simulink model "MMA"  (R2022a)
settings: Solver=VariableStepAuto  StartTime=0.0  StopTime=10.0  FixedStep=Ts  RelTol=1e-3
settings Model: Creator=juani  LastModifiedBy=juani

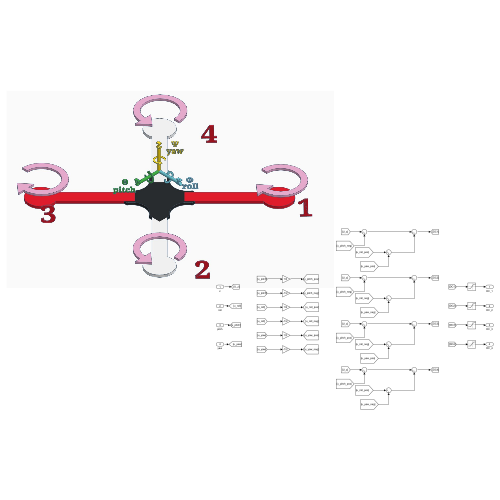
[thumbnail: Simulink's stored preview of the top-level diagram]
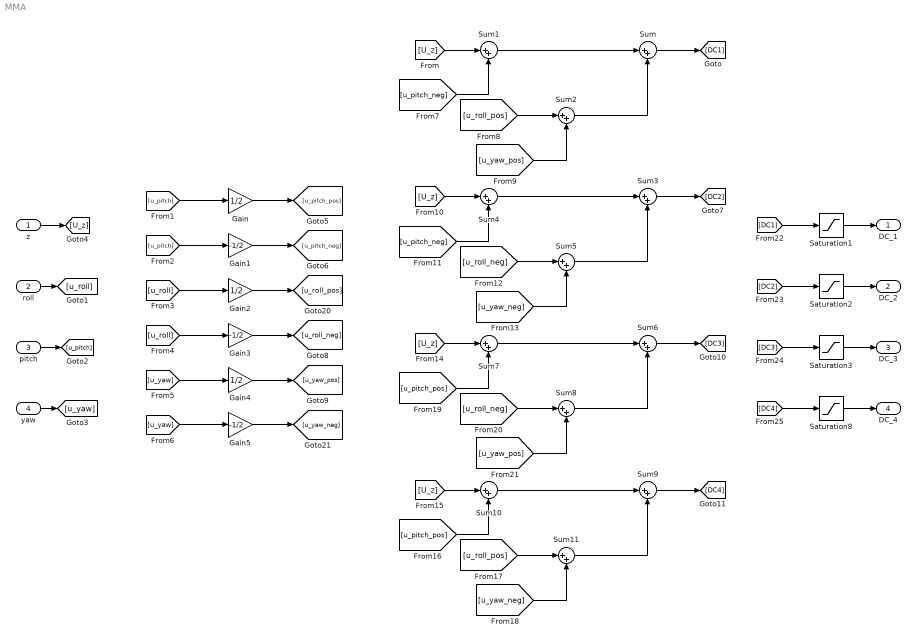
== system MMA ==
  z : Inport
  roll : Inport  Port=2
  pitch : Inport  Port=3
  yaw : Inport  Port=4
  Gain : Gain  Gain=1/2
  Gain1 : Gain  Gain=-1/2
  Gain2 : Gain  Gain=1/2
  Gain3 : Gain  Gain=-1/2
  Gain4 : Gain  Gain=1/2
  Gain5 : Gain  Gain=-1/2
  Saturation{1..3,8} (4 alike) : Saturate  UpperLimit=1  LowerLimit=0
  Sum{,1..11} (12 alike) : Sum  Inputs=|++
  DC_1 : Outport
  DC_2 : Outport  Port=2
  DC_3 : Outport  Port=3
  DC_4 : Outport  Port=4
  wires:
  yaw/1 -> [u_yaw]
  pitch/1 -> [u_pitch]
  roll/1 -> [u_roll]
  z/1 -> [U_z]
  [u_pitch] -> Gain/1
  [u_pitch] -> Gain1/1
  Gain/1 -> [u_pitch_pos]
  Gain1/1 -> [u_pitch_neg]
  [u_roll] -> Gain3/1
  Gain2/1 -> [u_roll_pos]
  [u_roll] -> Gain2/1
  Gain3/1 -> [u_roll_neg]
  [u_yaw] -> Gain4/1
  Gain5/1 -> [u_yaw_neg]
  Gain4/1 -> [u_yaw_pos]
  [u_yaw] -> Gain5/1
  Sum/1 -> [DC1]
  [U_z] -> Sum1/1
  [u_pitch_neg] -> Sum1/2
  Sum1/1 -> Sum/1
  [u_yaw_pos] -> Sum2/2
  [u_roll_pos] -> Sum2/1
  Sum2/1 -> Sum/2
  [u_pitch_neg] -> Sum4/2
  [u_roll_neg] -> Sum5/1
  Sum4/1 -> Sum3/1
  [u_yaw_neg] -> Sum5/2
  Sum3/1 -> [DC2]
  Sum5/1 -> Sum3/2
  [U_z] -> Sum4/1
  [u_pitch_pos] -> Sum7/2
  [u_roll_neg] -> Sum8/1
  [u_pitch_pos] -> Sum10/2
  [u_yaw_neg] -> Sum11/2
  [u_roll_pos] -> Sum11/1
  Sum10/1 -> Sum9/1
  Sum9/1 -> [DC4]
  Sum7/1 -> Sum6/1
  [u_yaw_pos] -> Sum8/2
  Sum11/1 -> Sum9/2
  Sum6/1 -> [DC3]
  Sum8/1 -> Sum6/2
  [U_z] -> Sum7/1
  [U_z] -> Sum10/1
  [DC2] -> Saturation2/1
  [DC3] -> Saturation3/1
  [DC1] -> Saturation1/1
  [DC4] -> Saturation8/1
  Saturation8/1 -> DC_4/1
  Saturation1/1 -> DC_1/1
  Saturation2/1 -> DC_2/1
  Saturation3/1 -> DC_3/1
